simulink model "lat_mpc"  (R2020b)
settings: Solver=FixedStepDiscrete  StartTime=0.0  StopTime=10.0  FixedStep=0.05  RelTol=1e-3
undefined symbols (not defined in the file): D
libraries: dspsolvers x2, dspfactors x1, dspsigattribs x1, dspmtrx3 x1
settings Model: Creator=chaoqun  LastModifiedBy=chaoqun
settings OptimizationCC: DefaultParameterBehavior=Inlined  EnhancedBackFolding=on  PassReuseOutputArgsAs=Individual arguments  ZeroExternalMemoryAtStartup=off  ZeroInternalMemoryAtStartup=off  OptimizeBlockOrder=speed  DifferentSizesBufferReuse=on  OptimizationCustomize=off  EfficientTunableParamExpr=on
settings DebuggingCC: ParameterTunabilityLossMsg=error
settings SFSimCC: MATLABDynamicMemAlloc=off
settings RTWCC: Description=Embedded Coder  SystemTargetFile=ert.tlc  GenCodeOnly=on  TemplateMakefile=ert_default_tmf
settings CodeAppCC: ForceParamTrailComments=on  IgnoreCustomStorageClasses=off  OperatorAnnotations=on  SimulinkDataObjDesc=on  SFDataObjDesc=on  InsertBlockDesc=on
settings ERTTargetCC: TargetLangStandard=C99 (ISO)  SupportVariableSizeSignals=on  InlinedParameterPlacement=NonHierarchical  ERTCustomFileTemplate=example_file_process.tlc

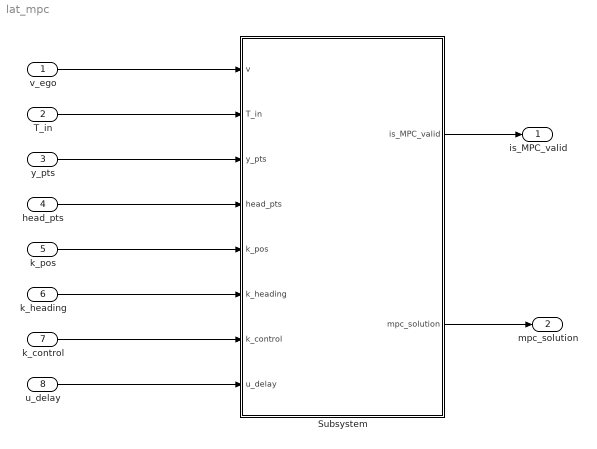
== system lat_mpc ==
  v_ego : Inport  OutDataTypeStr=single
  T_in : Inport  Port=2  OutDataTypeStr=single  PortDimensions=[1 30]
  y_pts : Inport  Port=3  OutDataTypeStr=single
  head_pts : Inport  Port=4  OutDataTypeStr=single
  k_pos : Inport  Port=5  OutDataTypeStr=single
  k_heading : Inport  Port=6  OutDataTypeStr=single
  k_control : Inport  Port=7  OutDataTypeStr=single
  u_delay : Inport  Port=8  OutDataTypeStr=single
  Subsystem : Subsystem
  is_MPC_valid : Outport  VectorParamsAs1DForOutWhenUnconnected=off
  mpc_solution : Outport  Port=2
  wires:
  Subsystem/1(is_MPC_valid) -> is_MPC_valid/1
  Subsystem/2(mpc_solution) -> mpc_solution/1
  v_ego/1 -> Subsystem/1(v)
  T_in/1 -> Subsystem/2(T_in)
  y_pts/1 -> Subsystem/3(y_pts)
  head_pts/1 -> Subsystem/4(head_pts)
  k_pos/1 -> Subsystem/5(k_pos)
  k_heading/1 -> Subsystem/6(k_heading)
  k_control/1 -> Subsystem/7(k_control)
  u_delay/1 -> Subsystem/8(u_delay)

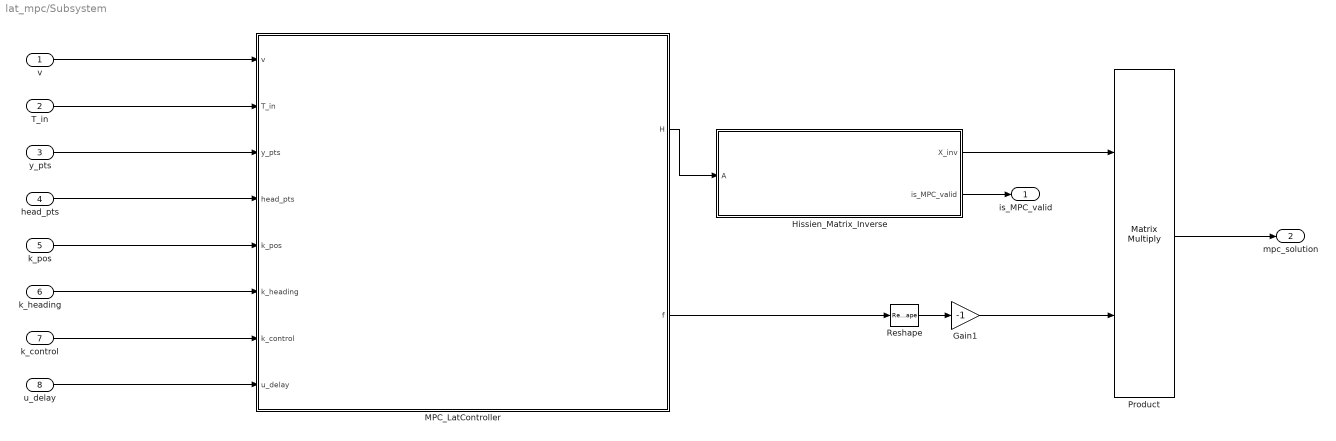
== system lat_mpc/Subsystem ==
  v : Inport
  T_in : Inport  Port=2
  y_pts : Inport  Port=3
  head_pts : Inport  Port=4
  k_pos : Inport  Port=5
  k_heading : Inport  Port=6
  k_control : Inport  Port=7
  u_delay : Inport  Port=8
  Gain1 : Gain  Gain=-1
  Hissien_Matrix_Inverse : Subsystem  AncestorBlock=dspinverses/ LU Inverse  mask(LU Inverse){}
      mask help: Matrix inverse using LU factorization.
      mask Help: eval('blocksethelp');
      mask Display:
      | text(0.25,0.85,'General')
      | text(0.25,0.70,'Inverse')
      | text(0.35,0.25,'(LU)')
  MPC_LatController : MATLAB Function  TreatAsAtomicUnit=on
  Product : Product  Inputs=**  Multiplication=Matrix(*)
  Reshape : Reshape  OutputDimensionality=Column vector (2-D)
  is_MPC_valid : Outport  VectorParamsAs1DForOutWhenUnconnected=off
  mpc_solution : Outport  Port=2
  wires:
  Hissien_Matrix_Inverse/1(X_inv) -> Product/1
  Hissien_Matrix_Inverse/2(is_MPC_valid) -> is_MPC_valid/1
  MPC_LatController/1(H) -> Hissien_Matrix_Inverse/1(A)
  Gain1/1 -> Product/2
  Reshape/1 -> Gain1/1
  y_pts/1 -> MPC_LatController/3(y_pts)
  head_pts/1 -> MPC_LatController/4(head_pts)
  Product/1 -> mpc_solution/1
  u_delay/1 -> MPC_LatController/8(u_delay)
  v/1 -> MPC_LatController/1(v)
  MPC_LatController/2(f) -> Reshape/1
  k_heading/1 -> MPC_LatController/6(k_heading)
  k_control/1 -> MPC_LatController/7(k_control)
  k_pos/1 -> MPC_LatController/5(k_pos)
  T_in/1 -> MPC_LatController/2(T_in)

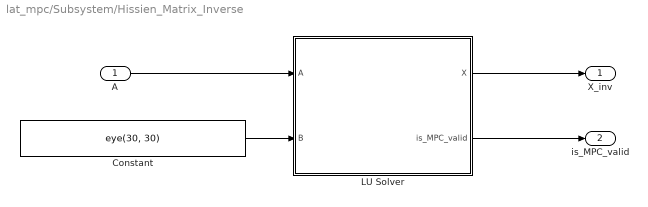
== system lat_mpc/Subsystem/Hissien_Matrix_Inverse ==
  A : Inport  OutDataTypeStr=single  PortDimensions=[30 30]
  Constant : Constant  Value=eye(30, 30)  OutDataTypeStr=single
  LU Solver : Subsystem  AncestorBlock=dspsolvers/LU Solver  mask(LU Solver){}
      mask help: dsp:dspsolvers:LUSolver_MD
      mask init:
      | x=[ 0.135 .475 0.475 0.135 .135 NaN 0.55 0.64 0.64 0.55 0.55 NaN 0.685 0.73 NaN 0.685 0.73 NaN 0.775 0.865 0.865 0.775 0.775 ];
      | y=[ 0.2 0.2 0.7 0.7 0.2 NaN 0.2 0.2 0.7 0.7 0.2 NaN 0.4 0.4 NaN 0.45 0.45 NaN 0.2 0.2 0.7 0.7 0.2 ];
      mask Help: eval('blocksethelp');
      mask Display:
      | plot(x,y+0.05);
      | 
      | text(0.25,0.9,'AX=B (LU)');
      | 
      | text(0.12,0.15,'[m x m]');
  X_inv : Outport  VectorParamsAs1DForOutWhenUnconnected=off
  is_MPC_valid : Outport  Port=2  VectorParamsAs1DForOutWhenUnconnected=off
  wires:
  A/1 -> LU Solver/1(A)
  LU Solver/1(X) -> X_inv/1
  LU Solver/2(is_MPC_valid) -> is_MPC_valid/1
  Constant/1 -> LU Solver/2(B)

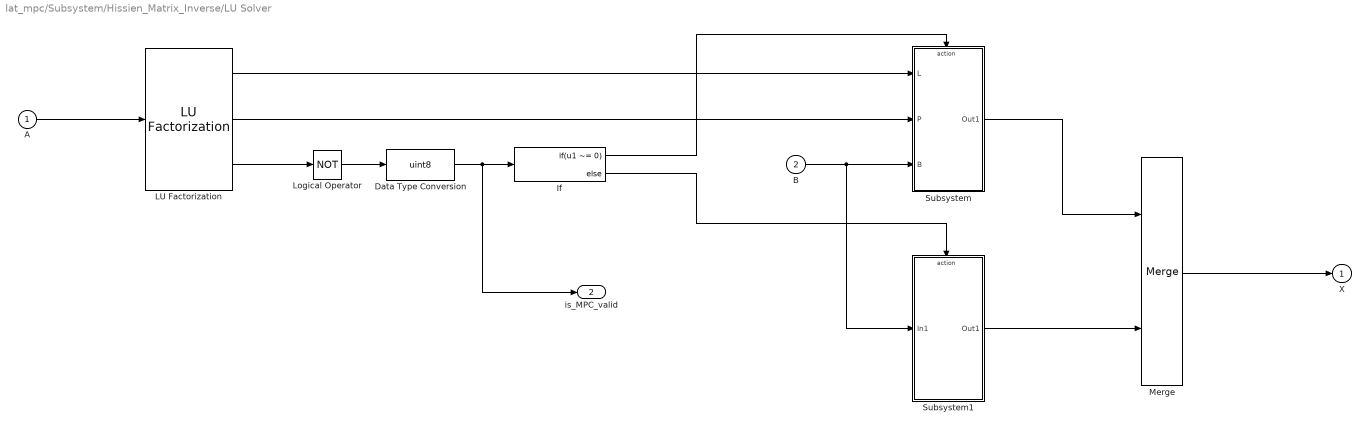
== system lat_mpc/Subsystem/Hissien_Matrix_Inverse/LU Solver ==
  A : Inport
  B : Inport  Port=2
  Data Type Conversion : DataTypeConversion  OutDataTypeStr=uint8
  If : If  IfExpression=u1 ~= 0
  LU Factorization : dspfactors/LU Factorization  singular=on  roundingMode=Floor  overflowMode=off  outputMin=[]  outputMax=[]
      settings: SourceProductBaseCode=DS
  Logical Operator : Logic  Operator=NOT  AllPortsSameDT=off  OutDataTypeStr=boolean
  Merge : Merge
  Subsystem : Subsystem
  Subsystem1 : Subsystem
  X : Outport  InitialOutput=0  VectorParamsAs1DForOutWhenUnconnected=off
  is_MPC_valid : Outport  Port=2  VectorParamsAs1DForOutWhenUnconnected=off
  wires:
  A/1 -> LU Factorization/1
  LU Factorization/1 -> Subsystem/1(L)
  LU Factorization/2 -> Subsystem/2(P)
  B/1 -> Subsystem1/1(In1), Subsystem/3(B)
  LU Factorization/3 -> Logical Operator/1
  Logical Operator/1 -> Data Type Conversion/1
  Data Type Conversion/1 -> is_MPC_valid/1, If/1
  If/1 -> Subsystem/Action
  If/2 -> Subsystem1/Action
  Subsystem1/1(Out1) -> Merge/2
  Subsystem/1(Out1) -> Merge/1
  Merge/1 -> X/1

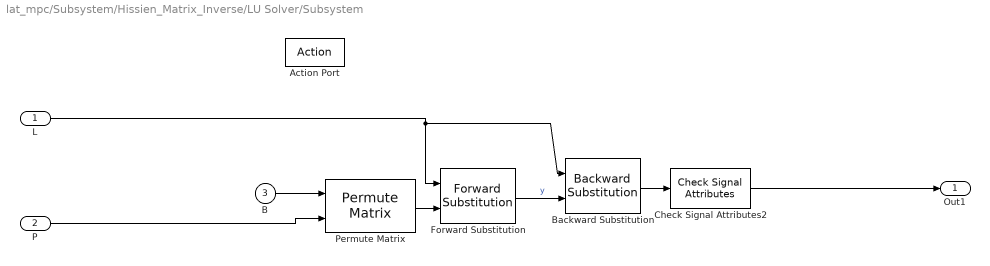
== system lat_mpc/Subsystem/Hissien_Matrix_Inverse/LU Solver/Subsystem ==
  L : Inport
  P : Inport  Port=2
  B : Inport  Port=3
  Action Port : ActionPort  ActionPortLabel=if(u1 ~= 0)
  Backward Substitution : dspsolvers/Backward Substitution  Unit=off  RealDiag=off  roundingMode=Floor  overflowMode=off  accumDataTypeStr=Inherit: Same as product output  accumLastDataTypeStr=Inherit: Same as product output  outputMin=[]  outputMax=[]
      settings: SourceProductBaseCode=DS
  Check Signal Attributes2 : dspsigattribs/Check Signal Attributes  SigAttribCheckMethod=Does not match attributes exactly  Complexity=Ignore  Frame=Ignore  DimsCheckMethod=Ignore  Dimensions=1-D  DatatypeCheckMethod=Is...  DatatypeGeneral=Floating-point  DtypeFloatSpecific=Any floating-point  DtypeFixedSpecific=Any fixed-point  DtypeIntSpecific=Any integer  SampleMode=Ignore
      settings: SourceProductBaseCode=DS
  Forward Substitution : dspsolvers/Forward Substitution  Unit=on  RealDiag=on  roundingMode=Floor  overflowMode=off  accumDataTypeStr=Inherit: Same as product output  accumLastDataTypeStr=Inherit: Same as product output  outputMin=[]  outputMax=[]
      settings: SourceProductBaseCode=DS
  Permute Matrix : dspmtrx3/Permute Matrix  mode=Rows  ZeroOneIdxMode=One-based  errmode=Clip index  checkDims=on
      settings: SourceProductBaseCode=DS
  Out1 : Outport  VectorParamsAs1DForOutWhenUnconnected=off
  wires:
  Backward Substitution/1 -> Check Signal Attributes2/1
  B/1 -> Permute Matrix/1
  P/1 -> Permute Matrix/2
  Check Signal Attributes2/1 -> Out1/1
  Forward Substitution/1 -> Backward Substitution/2  "y"
  L/1 -> Forward Substitution/1, Backward Substitution/1
  Permute Matrix/1 -> Forward Substitution/2

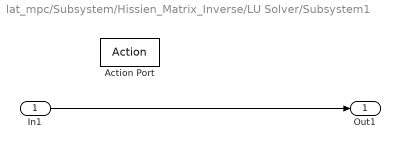
== system lat_mpc/Subsystem/Hissien_Matrix_Inverse/LU Solver/Subsystem1 ==
  In1 : Inport
  Action Port : ActionPort  ActionPortLabel=else
  Out1 : Outport  VectorParamsAs1DForOutWhenUnconnected=off
  wires:
  In1/1 -> Out1/1

== matlab function lat_mpc/Subsystem/MPC_LatController ==
  data: v input single; T_in input size=[1 30]; H output single; y_pts input single size=[1 30]; head_pts input single size=[1 30]; f output single; k_pos input; k_heading input; k_control input; u_delay input single size=[1 1]
function [H, f] = fcn(v, T_in, y_pts, head_pts, k_pos, k_heading, k_control, u_delay)

%% define controller parameters
p = 30;  % mpc predicted steps 
state_len = 3; % number of states


%% matrix initialization
% Q, R weight matrix 
Q = single(zeros(state_len*p, state_len*p)); 
R = single(k_control*eye(p)); 

% state transition matrix
A = single(zeros(3,3));
B = single(zeros(3,1));
A_ = single(zeros(3,3));
B_ = single(zeros(3,1));
A_set = single(zeros(p, 3, 3));
B_set = single(zeros(p, 3, 1));

% middle layer matrix
M = single(zeros(state_len*p, state_len));
K = single(zeros(state_len*p, p));

% reference desired state 
X_ref = single(zeros(state_len*p, 1));
yawrate_ref = single(zeros(p,1));
theta_ref = single(zeros(p,1));
y_ref = single(zeros(p, 1));

% QP solver matrix
H = single(zeros(p, p));
f = single(zeros(p, 1));

%% time array caculation
T =  T_in;

% referce x array
x_ref = v.*T;

%% intial states
x = single([0; 0; u_delay]); 


%% caculate X_ref, give the value for Q,R
% control input is delta of omiga
% matrix X_
%           |  y      | 
% X_ =	    |  theta  | 
%           |  omiga  | 

% matrix A_
%           |1    v*cos(theta)   0 | 
% A_ =	    |0    1             Ts | 
%           |0    0              1 | 

% matrix B_
%           |  0  | 
% B_ =	    |  0  | 
%           |  1  | 

% if X(k+1) = A*X(k) + B*u
% |X(k+1)|  | A   B | |X(k)|   |0|
%         =          *       + |0| * delta(u)
% |u(k+1)|  | 0   1 | |u(k)|   |1|

for i=1:p
    if i==1
        Ts = T(1);
    else
        Ts = T(i) - T(i-1);
    end

    % reference state
    x_tmp = x_ref(i);
    y_ref(i) = y_pts(i);
    theta_ref(i) = head_pts(i) ;
    yawrate_ref(i) = 0;
    X_ref((i-1)*state_len + 1:state_len*i, 1) = [y_ref(i) theta_ref(i) yawrate_ref(i) ];    
    
    % update A_, B_ set
    A_ = single([1 v*cos(theta_ref(i))*Ts; 0 1]);
    B_ = single([0 ; Ts]);

    A_set(i,:,:) = single([A_ B_; 0 0 1]);
    B_set(i,:,:) = single([0; 0 ;1]);
    
    % update Q weight matrix
    Q((i-1)*state_len + 1:state_len*i,  (i-1)*state_len + 1:state_len*i) = single([k_pos 0 0; 0 k_heading 0; 0 0 0]);

end

%% caculate M, K matrix
tmp_1 = single(eye(3));
tmp_2 = single(eye(3));

% M matrix update
% |  A1
% |  A2A1
% |  A3A2A1
% ..........

% K matrix update
% |0 0 0 ... 0            0         B1|
% |0 0 0 ... 0            A2B1  B2|
% |0 0 0 ... A3A2B1 A3B2  B3|
for i=1:p
   tmp_1 = reshape(A_set(i,:,:), [3 3])*tmp_1;
   M((i-1)*state_len + 1:state_len*i, 1:state_len) = tmp_1;

      for j=i:-1:1
        if j==i
            tmp_2 = single(eye(3));
        else
            tmp_2 = tmp_2*reshape(A_set(j+1,:,:), [3 3]);
        end
       K((i-1)*state_len + 1:state_len*i, j) = tmp_2*reshape(B_set(j,:,:), [3 1]);

      end
   
      
end

%% caculate H, f matrix for QP solver
X_pre = M*x;
E = X_pre - X_ref;

H = 2*(K'*Q*K + R);
f = (2*E'*Q*K)';

end

function prv_yawrate = preview_yawrate_calc(C1, C2, C3,C4, C5, d, v)
    ddy = 2*C2 + 6*C3*d + 12*C4*d^2 + 20*C5*d^3;
    
    dy = C1 + 2*C2*d + 3*C3*d^2+ 4*C4*d^3 +5*C5*d^4  ;
    
    prv_curve = ddy/((1+dy^2)^1.5);
    
    prv_yawrate = prv_curve * v;

end
